simulink model "TestFifo"  (Simulink 9.1)
settings: Solver=VariableStepAuto  StartTime=0.0  StopTime=100  RelTol=1e-3
InitFcn:
  | %% DSPBuilder Start
  | alt_dspbuilder_update_model(bdroot)
  | %% DSPBuilder End
StartFcn:
  | %% DSPBuilder Start
  | alt_dspbuilder_hdlimport_prepare_for_simulation(bdroot)
  | %% DSPBuilder End
libraries: allblocks_alteradspbuilder2 x1
settings Model: Creator=TungLT  LastModifiedBy=TungLT
settings DataIOCC: SaveFormat=Dataset
settings OptimizationCC: LifeSpan=auto
settings DebuggingCC: UnderspecifiedInitializationDetection=Simplified  MergeDetectMultiDrivingBlocksExec=error  SFUnexpectedBacktrackingDiag=error  SFNoUnconditionalDefaultTransitionDiag=error  SFExecutionAtInitializationDiag=warning
settings HardwareCC: ProdBitPerPointer=64  ProdBitPerSizeT=64  ProdBitPerPtrDiffT=64  ProdLargestAtomicFloat=Float  ProdIntDivRoundTo=Zero  ProdEndianess=LittleEndian  ProdWordSize=64  ProdHWDeviceType=Intel->x86-64 (Windows64)
settings ModelReferenceCC: PropagateSignalLabelsOutOfModel=on
settings CodeAppCC: StateflowObjectComments=off
settings GRTTargetCC: TargetLangStandard=C99 (ISO)  CombineOutputUpdateFcns=on  GRTInterface=off
settings ConfigComp: CovMetricSettings=dwe  CovHtmlReporting=off  CovSaveCumulativeToWorkspaceVar=off  CovSaveSingleToWorkspaceVar=off  CovExternalEMLEnable=on

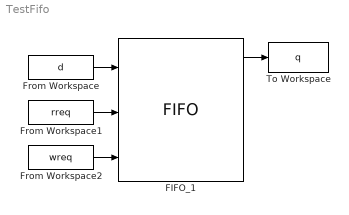
== system TestFifo ==
  FIFO_1 : allblocks_alteradspbuilder2/FIFO  numwords=1024  BusType=Unsigned Integer  bwl=8  bwr=0  ram_type=AUTO  use_sclr=off  use_les_only=off  showahead_mode=off  allowFloatingPointOverride=on  logOutputs=off  logFile=C:\TestFifo_FIFO%5F1%3A%3Aq.fixedpointlog,C:\TestFifo_FIFO%5F1%3A%3Afull.fixedpointlog,C:\TestFifo_FIFO%5F1%3A%3Aempty.fixedpointlog,C:\TestFifo_FIFO%5F1%3A%3Ausedw.fixedpointlog,
  From Workspace : FromWorkspace  VariableName=d  SampleTime=0
  From Workspace1 : FromWorkspace  VariableName=rreq  SampleTime=0
  From Workspace2 : FromWorkspace  VariableName=wreq  SampleTime=0
  To Workspace : ToWorkspace  VariableName=q  SampleTime=-1
      settings: Save2DSignal=2-D array (concatenate along first dimension)
  wires:
  From Workspace/1 -> FIFO_1/1
  FIFO_1/1 -> To Workspace/1
  From Workspace1/1 -> FIFO_1/2
  From Workspace2/1 -> FIFO_1/3
